simulink model "bengji_sfunction"  (R2021a)
settings: Solver=FixedStepAuto  StartTime=0.0  StopTime=50.0  FixedStep=0.1  RelTol=1e-3
model workspace (MAT data in the model file):
  times = 1
settings Model: Creator=86137  LastModifiedBy=86137

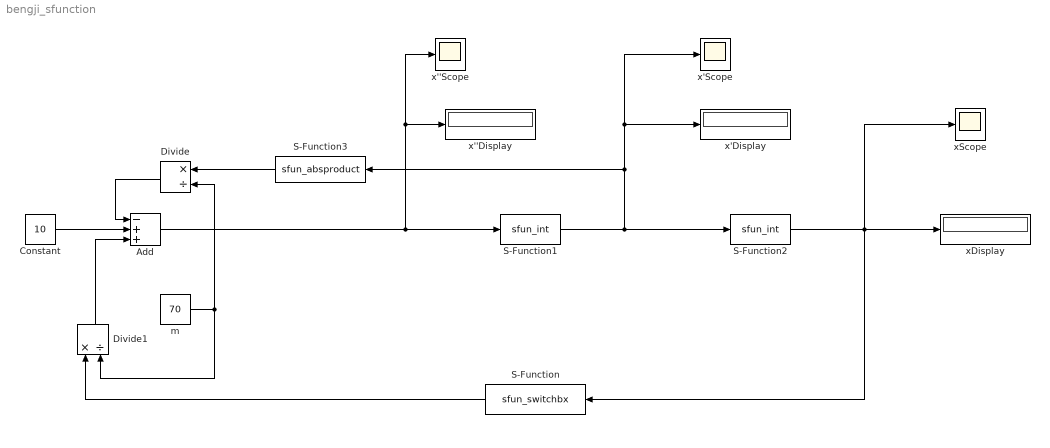
== system bengji_sfunction ==
  Add : Sum  Inputs=-++
  Constant : Constant  Value=10
  Divide : Product  Inputs=*/
  Divide1 : Product  Inputs=*/
  S-Function : S-Function  FunctionName=sfun_switchbx  SFunctionDeploymentMode=off  EnableBusSupport=off
  S-Function1 : S-Function  FunctionName=sfun_int  Parameters=0  SFunctionDeploymentMode=off  EnableBusSupport=off
  S-Function2 : S-Function  FunctionName=sfun_int  Parameters=-30  SFunctionDeploymentMode=off  EnableBusSupport=off
  S-Function3 : S-Function  FunctionName=sfun_absproduct  SFunctionDeploymentMode=off  EnableBusSupport=off
  m : Constant  Value=70
  x''Display : Display
  x''Scope : Scope
  x'Display : Display
  x'Scope : Scope
  xDisplay : Display
  xScope : Scope
  wires:
  Constant/1 -> Add/2
  Add/1 -> S-Function1/1, x''Display/1, x''Scope/1
  S-Function3/1 -> Divide/1
  Divide/1 -> Add/1
  m/1 -> Divide1/2, Divide/2
  S-Function2/1 -> S-Function/1, xScope/1, xDisplay/1
  Divide1/1 -> Add/3
  S-Function1/1 -> S-Function2/1, S-Function3/1, x'Scope/1, x'Display/1
  S-Function/1 -> Divide1/1
